simulink model "simulacion_ROS"  (R2025b)
settings: Solver=ode14x  StartTime=0.0  StopTime=20  FixedStep=0.01  RelTol=1e-3
InitFcn:
  | start_time_epoch = posixtime(datetime('now'))-3600;
  | setenv('ROS_LOCALHOST_ONLY', '');
  | setenv('RMW_IMPLEMENTATION','rmw_cyclonedds_cpp')
values from neighbouring files (symbols this model uses):
  A = [zeros(2),        eye(2) ... (first row only)    [parametros_planta.m]
  B = [0;0;[M_bar\[1;0]]]    [parametros_planta.m]
  cc = 0.05    [parametros_planta.m]
  cp = 0.0005    [parametros_planta.m]
  g = 9.81    [parametros_planta.m]
  J = 0.0136    [parametros_planta.m]
  lcm = 0.17    [parametros_planta.m]
  M = mp + mc    (= 1.23)    [parametros_planta.m]
  mc = 1.12    [parametros_planta.m]
  mp = 0.11    [parametros_planta.m]
undefined symbols (not defined in the file or in its folder): K_lqr
libraries: ros2lib x2
settings Model: Creator=miguel  LastModifiedBy=miguel
settings SolverCC: EnableFixedStepZeroCrossing=on
settings OptimizationCC: DefaultParameterBehavior=Inlined  EnhancedBackFolding=on  PassReuseOutputArgsAs=Individual arguments  ZeroExternalMemoryAtStartup=off  ZeroInternalMemoryAtStartup=off  MaxStackSize=64  OptimizeBlockOrder=speed  DifferentSizesBufferReuse=on  OptimizationCustomize=off  EfficientTunableParamExpr=on
settings DebuggingCC: ParameterTunabilityLossMsg=error
settings HardwareCC: ProdBitPerLong=64.0  ProdHWDeviceType=Intel->x86-64 (Linux 64)  UseEmbeddedCoderFeatures=off
settings SFSimCC: MATLABDynamicMemAlloc=off
settings RTWCC: SystemTargetFile=ert.tlc  HardwareBoard=Robot Operating System 2 (ROS 2)  TLCOptions="-aInlineSetEventsForThisBaseRateFcn=TLC_FALSE -aSuppressMultiTaskScheduler=TLC_FALSE  -aRateBasedStepFcn=0"  TemplateMakefile=ert_default_tmf  Toolchain=Colcon Tools  TargetLang=C++  Description=Embedded Coder
settings CodeAppCC: ForceParamTrailComments=on  IgnoreCustomStorageClasses=off  OperatorAnnotations=on  SimulinkDataObjDesc=on  SFDataObjDesc=on  InsertBlockDesc=on
settings ERTTargetCC: ExtModeTransport=2.0  ExtModeStaticAlloc=on  ExtModeAutomaticAllocSize=off  ExtModeMexFile=ext_xcp  ExtModeIntrfLevel=Level2 - Open  RootIOFormat=Structure reference  CodeInterfacePackaging=C++ class  SupportNonInlinedSFcns=on

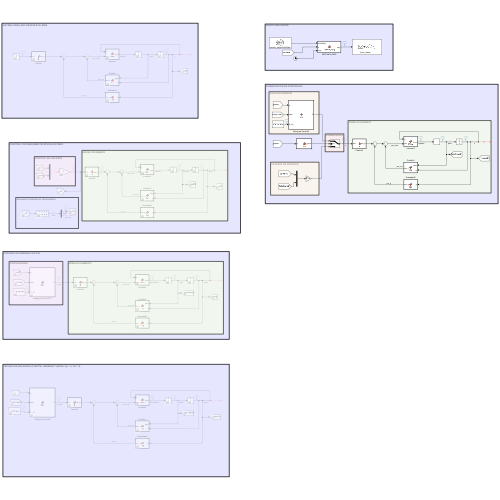
[thumbnail: Simulink's stored preview of the top-level diagram]
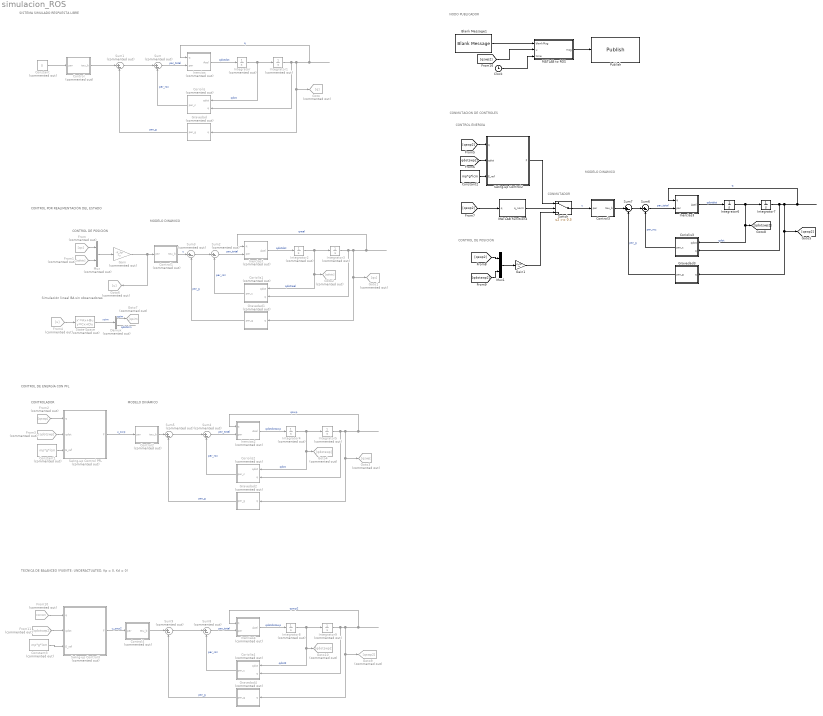
== system simulacion_ROS ==
  note: CONTROLADOR
  note: MODELO DINÁMICO
  note: CONTROL DE POSICIÓN
  note: MODELO DINÁMICO
  note: CONMUTADOR
  note: MODELO DINÁMICO
  note: CONTROL ENERGÍA
  note: CONTROL DE POSICIÓN
  note: Simulación lineal BA sin observadores
  note: SISTEMA SIMULADO RESPUESTA LIBRE
  note: NODO PUBLICADOR
  note: CONTROL POR REALIMENTACIÓN DEL ESTADO
  note: CONTROL DE ENERGÍA CON PFL
  note: CONMUTACION DE CONTROLES
  note: TECNICA DE BALANCEO (FUENTE: UNDERACTUATED, Kp = 0, Kd = 0)
  Blank Message1 : ros2lib/Blank Message  messageClass=Message  entityType=sensor_msgs/JointState  messageType=sensor_msgs/JointState  SampleTime=inf
  Clock : Clock
  Constant : Constant  Commented=on  Value=0
  Constant1 : Constant  Commented=on  Value=mp*g*lcm
  Constant2 : Constant  Value=mp*g*lcm
  Constant3 : Constant  Commented=on  Value=mp*g*lcm
  Control : MATLAB Function  Commented=on  TreatAsAtomicUnit=on
  Control1 : MATLAB Function  Commented=on  TreatAsAtomicUnit=on
  Control2 : MATLAB Function  Commented=on  TreatAsAtomicUnit=on
  Control3 : MATLAB Function  TreatAsAtomicUnit=on
  Control4 : MATLAB Function  Commented=on  TreatAsAtomicUnit=on
  Coriolis : MATLAB Function  Commented=on  TreatAsAtomicUnit=on
  Coriolis1 : MATLAB Function  Commented=on  TreatAsAtomicUnit=on
  Coriolis2 : MATLAB Function  Commented=on  TreatAsAtomicUnit=on
  Coriolis3 : MATLAB Function  TreatAsAtomicUnit=on
  Coriolis4 : MATLAB Function  Commented=on  TreatAsAtomicUnit=on
  Demux : Demux  Commented=on  Outputs=2
  From : From  Commented=on  GotoTag=qc
  From1 : From  Commented=on  GotoTag=qdotc
  From10 : From  Commented=on  GotoTag=qswp2
  From11 : From  Commented=on  GotoTag=qdotswp2
  From2 : From  Commented=on  GotoTag=qswp
  From3 : From  Commented=on  GotoTag=qdotswp
  From4 : From  Commented=on  GotoTag=u
  Gain : Gain  Commented=on  Gain=-K_lqr  Multiplication=Matrix(K*u)
  Gain1 : Gain  Gain=-K_lqr  Multiplication=Matrix(K*u)
  Goto : Goto  Commented=on  GotoTag=q
  Goto1 : Goto  Commented=on  GotoTag=qc
  Goto10 : Goto  Commented=on  GotoTag=qdotswp2
  Goto2 : Goto  Commented=on  GotoTag=qdotc
  Goto3 : Goto  Commented=on  GotoTag=qswp
  Goto4 : Goto  Commented=on  GotoTag=qdotswp
  Goto6 : Goto  Commented=on  GotoTag=u
  Goto7 : Goto  Commented=on  GotoTag=qsim
  Goto9 : Goto  Commented=on  GotoTag=qswp2
  Gravedad : MATLAB Function  Commented=on  TreatAsAtomicUnit=on
  Gravedad1 : MATLAB Function  Commented=on  TreatAsAtomicUnit=on
  Gravedad2 : MATLAB Function  Commented=on  TreatAsAtomicUnit=on
  Gravedad3 : MATLAB Function  TreatAsAtomicUnit=on
  Gravedad4 : MATLAB Function  Commented=on  TreatAsAtomicUnit=on
  Inercias : MATLAB Function  Commented=on  TreatAsAtomicUnit=on
  Inercias1 : MATLAB Function  Commented=on  TreatAsAtomicUnit=on
  Inercias2 : MATLAB Function  Commented=on  TreatAsAtomicUnit=on
  Inercias3 : MATLAB Function  TreatAsAtomicUnit=on
  Inercias4 : MATLAB Function  Commented=on  TreatAsAtomicUnit=on
  Integrator : Integrator  Commented=on  InitialCondition=[0; 0]
  Integrator1 : Integrator  Commented=on  InitialCondition=[0; 0.1]
  Integrator2 : Integrator  Commented=on  InitialCondition=[0; 0]
  Integrator3 : Integrator  Commented=on  InitialCondition=[0; 0.2]
  Integrator4 : Integrator  Commented=on  InitialCondition=[0; 0.01]
  Integrator5 : Integrator  Commented=on  InitialCondition=[0; 3.14]
  Integrator6 : Integrator  InitialCondition=[0; 0.01]
  Integrator7 : Integrator  InitialCondition=[0; 3.14]
  Integrator8 : Integrator  Commented=on  InitialCondition=[0; 0.01]
  Integrator9 : Integrator  Commented=on  InitialCondition=[0; 3.14]
  MATLAB Function4 : MATLAB Function  TreatAsAtomicUnit=on
  MATLAB to ROS : MATLAB Function  TreatAsAtomicUnit=on
  Mux : Mux  Commented=on  Inputs=2
  Mux1 : Mux  Inputs=2
  Publish : ros2lib/Publish  topicSource=Specify your own  topic=/joint_states  messageType=sensor_msgs/JointState  QOSHistory=Keep last  QOSDepth=10  QOSReliability=Reliable  QOSDurability=Volatile  QOSDeadline=Inf  QOSLifespan=Inf  QOSLiveliness=Automatic  QOSLeaseDuration=Inf  QOSAvoidROSNamespaceConventions=off
  State-Space : StateSpace  Commented=on  A=A  B=B  C=eye(4)  D=[0; 0; 0; 0]  InitialCondition=[0; 0.2; 0; 0]
  Sum{,1..5,8..9} (8 alike) : Sum  Commented=on  Inputs=|+-
  Sum6 : Sum  Inputs=|+-
  Sum7 : Sum  Inputs=|+-
  Swing-up Control PFL : MATLAB Function  Commented=on  TreatAsAtomicUnit=on
  Swing-up Control2 : MATLAB Function  TreatAsAtomicUnit=on
  Swing-up Control3 : MATLAB Function  Commented=on  TreatAsAtomicUnit=on
  Switch : Switch  Threshold=0.3  SaturateOnIntegerOverflow=off  InputSameDT=off
  wires:
  Sum1/1 -> Sum/1
  Gravedad/1(par_g) -> Sum1/2  "par_g"
  Control/1(tau_b) -> Sum1/1
  Integrator1/1 -> Coriolis/2(q), Goto/1, Gravedad/1(q), Inercias/1(q)  "q"
  Inercias/1(Acel) -> Integrator/1  "qdotdot"
  Constant/1 -> Control/1(par)
  Integrator/1 -> Coriolis/1(qdot), Integrator1/1  "qdot"
  Sum/1 -> Inercias/2(par)  "par_total"
  Coriolis/1(par_c) -> Sum/2  "par_roz"
  Blank Message1/1 -> MATLAB to ROS/1(blankMsg)
  MATLAB to ROS/1(msg) -> Publish/1
  Clock/1 -> MATLAB to ROS/3(time)
  [qswp2] -> MATLAB to ROS/2(u)
  Coriolis1/1(par_c) -> Sum2/2  "par_roz"
  Control1/1(tau_b) -> Sum3/1  "u"
  Integrator3/1 -> Coriolis1/2(q), Goto1/1, Gravedad1/1(q), Inercias1/1(q)  "qreal"
  Inercias1/1(Acel) -> Integrator2/1  "qdotdot"
  Sum2/1 -> Inercias1/2(par)  "par_total"
  Gravedad1/1(par_g) -> Sum3/2  "par_g"
  Sum3/1 -> Sum2/1
  Integrator2/1 -> Goto2/1, Coriolis1/1(qdot), Integrator3/1  "qdotreal"
  Mux/1 -> Gain/1
  From/1 -> Mux/1
  From1/1 -> Mux/2
  From4/1 -> State-Space/1
  State-Space/1 -> Demux/1  "xsim"
  Demux/1 -> Goto7/1  "qsim"
  Demux/2 -> ?  "qdotsim"
  Inercias2/1(Acel) -> Integrator4/1  "qdotdotswp"
  Integrator5/1 -> Coriolis2/2(q), Goto3/1, Gravedad2/1(q), Inercias2/1(q)  "qswp"
  Sum5/1 -> Sum4/1
  Gravedad2/1(par_g) -> Sum5/2  "par_g"
  Control2/1(tau_b) -> Sum5/1
  Integrator4/1 -> Goto4/1, Coriolis2/1(qdot), Integrator5/1  "qdot"
  Sum4/1 -> Inercias2/2(par)  "par_total"
  Coriolis2/1(par_c) -> Sum4/2  "par_roz"
  Swing-up Control PFL/1(F) -> Control2/1(par)  "u_swp"
  From2/1 -> Swing-up Control PFL/1(q)
  From3/1 -> Swing-up Control PFL/2(qdot)
  Constant2/1 -> Swing-up Control2/3(E_ref)
  Control3/1(tau_b) -> Sum7/1
  Coriolis3/1(par_c) -> Sum6/2  "par_roz"
  Sum7/1 -> Sum6/1
  Inercias3/1(Acel) -> Integrator6/1  "qdotdot"
  [qdotswp2] -> Swing-up Control2/2(qdot)
  Integrator6/1 -> [qdotswp2], Coriolis3/1(qdot), Integrator7/1  "qdot"
  Sum6/1 -> Inercias3/2(par)  "par_total"
  [qswp2] -> Swing-up Control2/1(q)
  Gravedad3/1(par_g) -> Sum7/2  "par_g"
  Integrator7/1 -> Coriolis3/2(q), [qswp2], Gravedad3/1(q), Inercias3/1(q)  "q"
  Switch/1 -> Control3/1(par)  "u"
  Swing-up Control2/1(F) -> Switch/1
  MATLAB Function4/1(q_norm) -> Switch/2
  [qswp2] -> MATLAB Function4/1(q)
  [qswp2] -> Mux1/1
  Mux1/1 -> Gain1/1
  [qdotswp2] -> Mux1/2
  Gain1/1 -> Switch/3
  Constant3/1 -> Swing-up Control3/3(E_ref)
  Control4/1(tau_b) -> Sum9/1
  Coriolis4/1(par_c) -> Sum8/2  "par_roz"
  Sum9/1 -> Sum8/1
  Inercias4/1(Acel) -> Integrator8/1  "qdotdotswp"
  From11/1 -> Swing-up Control3/2(qdot)
  Integrator8/1 -> Goto10/1, Coriolis4/1(qdot), Integrator9/1  "qdot2"
  Swing-up Control3/1(F) -> Control4/1(par)  "u_swp2"
  Sum8/1 -> Inercias4/2(par)  "par_total"
  From10/1 -> Swing-up Control3/1(q)
  Gravedad4/1(par_g) -> Sum9/2  "par_g"
  Integrator9/1 -> Coriolis4/2(q), Goto9/1, Gravedad4/1(q), Inercias4/1(q)  "qswp2"
  Constant1/1 -> Swing-up Control PFL/3(E_ref)
  Gain/1 -> Goto6/1, Control1/1(par)

== matlab function simulacion_ROS/Control2 ==
  data: par input; tau_b output
function tau_b = B(par)

tau_b = [1; 0]*par; %Nuestra acción de control se aplica sobre el eje horizontal.

== matlab function simulacion_ROS/Coriolis2 ==
  data: qdot input; q input; par_c output size=[2, 1]; cc parameter; cp parameter; mp parameter; lcm parameter
function par_c = Cq(qdot, q, cc, cp, mp, lcm)

%Nota: cp = 0 Nm.rad/s no me lo creo habrá que estimarlo de forma
%conservadora.

C = [cc,   -mp*lcm*qdot(2)*sin(q(2))
      0,          cp        ]; 

par_c = C*qdot;

== matlab function simulacion_ROS/Gravedad2 ==
  data: q input; par_g output; mp parameter; g parameter; lcm parameter
function par_g = Gq(q, mp, g, lcm)
G = [0; -mp*g*lcm*sin(q(2))]; 

par_g = G;

== matlab function simulacion_ROS/Inercias2 ==
  data: q input; par input; Acel output; J parameter; M parameter; mp parameter; lcm parameter
function Acel = Minv(q,par, J, M, mp, lcm)
%La matriz va aumentando su dimensionalidad a medida que se añaden GDLs

M = [M,          +mp*lcm*cos(q(2));
    +mp*lcm*cos(q(2)),      J]; 

Acel = M\par; %División de matrices.

== matlab function simulacion_ROS/Control3 ==
  data: par input; tau_b output
function tau_b = B(par)

tau_b = [1; 0]*par; %Nuestra acción de control se aplica sobre el eje horizontal.

== matlab function simulacion_ROS/Swing-up Control PFL ==
  data: q input; F output; qdot input; E_ref input; mp parameter; lcm parameter; cp parameter; cc parameter; J parameter; mc parameter
function F = fcn(q, qdot, E_ref, mp, lcm, cp, cc, J, mc) % Añadido Mc y salida F

% --- PARAMETROS FISICOS Y GANANCIAS ---
g = 9.81; % Añadido el punto y coma

% Ganancias del control de energía (Swing-up) AJUSTAR
Ke = 26; 
kp = 8.16; 
kd = 4; 

% -- ESTADOS DEL SISTEMA --
x = q(1);        % Posición del carro
theta = q(2);    % Ángulo del péndulo (0 = arriba)
xdot = qdot(1);  % Velocidad del carro
thetadot = qdot(2); % Velocidad angular

% --- 1. CÁLCULO DE ENERGÍA ---
Ep = mp * g * lcm * cos(theta); 
Ek = 0.5 * J * thetadot^2;
E_total = Ep + Ek;

% --- 2. LEY DE CONTROL DE ENERGÍA (Aceleración 'u') ---
e = E_total - E_ref;
u = Ke * thetadot * cos(theta) * e - kp * x - kd * xdot;

% --- 3. LINEARIZACIÓN POR RETROALIMENTACIÓN PARCIAL (PFL) ---
% Convierte la aceleración deseada 'u' en Fuerza 'F' para el motor

thetadotdot = 1/J *(-mp*lcm*cos(theta)*u ...
    + mp*g*lcm*sin(theta) -cp*thetadot);

F = (mc + mp) * u ...
    - (mp * lcm * thetadot^2 * sin(theta)) ...
    + (mp * lcm * cos(theta)) * thetadotdot ...
    +cc*xdot;

%Saturacion --> Evitar oscilaciones iniciales bruscas.
F_max = 2; % Newtons
if F > F_max
    F = F_max;
elseif F < -F_max
    F = -F_max;
end

end

== matlab function simulacion_ROS/Coriolis3 ==
  data: qdot input; q input; par_c output size=[2, 1]; cc parameter; cp parameter; mp parameter; lcm parameter
function par_c = Cq(qdot, q, cc, cp, mp, lcm)

%Nota: cp = 0 Nm.rad/s no me lo creo habrá que estimarlo de forma
%conservadora.

C = [cc,   -mp*lcm*qdot(2)*sin(q(2))
      0,          cp        ]; 

par_c = C*qdot;

== matlab function simulacion_ROS/Gravedad3 ==
  data: q input; par_g output; mp parameter; g parameter; lcm parameter
function par_g = Gq(q, mp, g, lcm)
G = [0; -mp*g*lcm*sin(q(2))]; 

par_g = G;

== matlab function simulacion_ROS/Inercias3 ==
  data: q input; par input; Acel output; J parameter; M parameter; mp parameter; lcm parameter
function Acel = Minv(q,par, J, M, mp, lcm)
%La matriz va aumentando su dimensionalidad a medida que se añaden GDLs

M = [M,          +mp*lcm*cos(q(2));
    +mp*lcm*cos(q(2)),      J]; 

Acel = M\par; %División de matrices.

== matlab function simulacion_ROS/Swing-up Control2 ==
  data: q input; F output; qdot input; E_ref input; mp parameter; lcm parameter; cp parameter; cc parameter; J parameter; mc parameter
function F = fcn(q, qdot, E_ref, mp, lcm, cp, cc, J, mc) 

% --- PARAMETROS FISICOS Y GANANCIAS ---
g = 9.81; 

% Ganancias del control de energía (Swing-up)
Ke = 26; 
kp = 6; 
kd = 4; 

% -- ESTADOS DEL SISTEMA --
x = q(1);        % Posición del carro
theta = q(2);    % Ángulo del péndulo 
xdot = qdot(1);  % Velocidad del carro
thetadot = qdot(2); % Velocidad angular

% --- 1. CÁLCULO DE ENERGÍA ---
Ep = mp * g * lcm * cos(theta); 
Ek = 0.5 * J * thetadot^2;
E_total = Ep + Ek;

% --- 2. LEY DE CONTROL DE ENERGÍA (Aceleración 'u') ---
e = E_total - E_ref;
u = Ke * thetadot * cos(theta) * e - kp * x - kd * xdot;

% --- 3. LINEARIZACIÓN POR RETROALIMENTACIÓN PARCIAL (PFL) ---
% Convierte la aceleración deseada 'u' en Fuerza 'F' para el motor

thetadotdot = 1/J *(-mp*lcm*cos(theta)*u ...
    + mp*g*lcm*sin(theta) -cp*thetadot);

F = (mc + mp) * u ...
    - (mp * lcm * thetadot^2 * sin(theta)) ...
    + (mp * lcm * cos(theta)) * thetadotdot ...
    +cc*xdot;

%Saturacion --> Evitar oscilaciones iniciales bruscas.
F_max = 2; % Newtons
if F > F_max
    F = F_max;
elseif F < -F_max
    F = -F_max;
end

end

== matlab function simulacion_ROS/Coriolis ==
  data: qdot input; q input; par_c output size=[2, 1]; cc parameter; cp parameter; mp parameter; lcm parameter
function par_c = Cq(qdot, q, cc, cp, mp, lcm)

%Nota: cp = 0 Nm.rad/s no me lo creo habrá que estimarlo de forma
%conservadora.

C = [cc,   -mp*lcm*qdot(2)*sin(q(2))
      0,          cp        ]; 

par_c = C*qdot;

== matlab function simulacion_ROS/MATLAB Function4 ==
  data: q input; q_norm output
function q_norm = fcn(q)
    % Esto envuelve el ángulo para que siempre esté entre -pi y +pi
    q_norm = atan2(sin(q(2)), cos(q(2)));
    q_norm = abs(q_norm);
end

== matlab function simulacion_ROS/MATLAB to ROS ==
  data: blankMsg input; msg output Bus: SL_Bus_sensor_msgs_JointState; u input; time input; start_time_epoch parameter
function msg = create_msg(blankMsg, u, time, start_time_epoch)
%#codegen
msg = blankMsg;

%Sincronización con el reloj interno de la máquina.
total_time = start_time_epoch + time; 
%Indicar el tiempo de simulación para que RViz pueda componer la
%simulación. 
s = floor(total_time);
ns = (total_time - s) * 1e9;  
msg.header.stamp.sec = int32(s);
msg.header.stamp.nanosec = uint32(ns);

% Definimos los nombres y sus posiciones correspondientes
strArrayToAssign = {'cart_slider', 'pole_joint'};
% Las posiciones angulares de nuestro péndulo. 
positionsToAssign = [u(1), u(2)]; 

% 1. Configurar NOMBRES (Strings)
numStringsInArray = length(strArrayToAssign);
msg.name_SL_Info.CurrentLength = uint32(numStringsInArray);

for idx=1:numStringsInArray
    str = strArrayToAssign{idx};
    strLength = length(str);
    % Asignar caracteres convertidos a uint8
    msg.name(idx).data(1:strLength) = uint8(str);
    msg.name(idx).data_SL_Info.CurrentLength = uint32(strLength);
end

% 2. Configurar POSICIONES (float64 array)
% El campo 'position' en un Bus de Simulink para JointState 
% también tiene un campo _SL_Info asociado para controlar la longitud.
numPositions = length(positionsToAssign);
msg.position_SL_Info.CurrentLength = uint32(numPositions);
% Asignamos los valores directamente
msg.position(1:numPositions) = positionsToAssign;

% 3. Dejar sin campo de velocidad y esfuerzo el tópico.
msg.velocity_SL_Info.CurrentLength = uint32(0);
msg.effort_SL_Info.CurrentLength = uint32(0);

end

== matlab function simulacion_ROS/Control4 ==
  data: par input; tau_b output
function tau_b = B(par)

tau_b = [1; 0]*par; %Nuestra acción de control se aplica sobre el eje horizontal.

== matlab function simulacion_ROS/Coriolis4 ==
  data: qdot input; q input; par_c output size=[2, 1]; cc parameter; cp parameter; mp parameter; lcm parameter
function par_c = Cq(qdot, q, cc, cp, mp, lcm)

%Nota: cp = 0 Nm.rad/s no me lo creo habrá que estimarlo de forma
%conservadora.

C = [cc,   -mp*lcm*qdot(2)*sin(q(2))
      0,          cp        ]; 

par_c = C*qdot;

== matlab function simulacion_ROS/Gravedad4 ==
  data: q input; par_g output; mp parameter; g parameter; lcm parameter
function par_g = Gq(q, mp, g, lcm)
G = [0; -mp*g*lcm*sin(q(2))]; 

par_g = G;

== matlab function simulacion_ROS/Inercias4 ==
  data: q input; par input; Acel output; J parameter; M parameter; mp parameter; lcm parameter
function Acel = Minv(q,par, J, M, mp, lcm)
%La matriz va aumentando su dimensionalidad a medida que se añaden GDLs

M = [M,          +mp*lcm*cos(q(2));
    +mp*lcm*cos(q(2)),      J]; 

Acel = M\par; %División de matrices.

== matlab function simulacion_ROS/Swing-up Control3 ==
  data: q input; F output; qdot input; E_ref input; mp parameter; lcm parameter; cp parameter; cc parameter; J parameter; mc parameter
function F = fcn(q, qdot, E_ref, mp, lcm, cp, cc, J, mc) % Añadido Mc y salida F

% --- PARAMETROS FISICOS Y GANANCIAS ---
g = 9.81; % Añadido el punto y coma

% Ganancias del control de energía (Swing-up) AJUSTAR
Ke = 4; 
kp = 1.77; 
kd = 2.66; 

% -- ESTADOS DEL SISTEMA --
x = q(1);        % Posición del carro
theta = q(2);    % Ángulo del péndulo (0 = arriba)
xdot = qdot(1);  % Velocidad del carro
thetadot = qdot(2); % Velocidad angular

% --- 1. CÁLCULO DE ENERGÍA ---
Ep = mp * g * lcm * cos(theta); 
Ek = 0.5 * J * thetadot^2;
E_total = Ep + Ek;

% --- 2. LEY DE CONTROL DE ENERGÍA (Aceleración 'u') ---
e = E_total - E_ref;
u = Ke * thetadot * cos(theta) * e ;%- kp * x - kd * xdot;

% --- 3. LINEARIZACIÓN POR RETROALIMENTACIÓN PARCIAL (PFL) ---
% Convierte la aceleración deseada 'u' en Fuerza 'F' para el motor

thetadotdot = 1/J *(-mp*lcm*cos(theta)*u ...
    + mp*g*lcm*sin(theta) -cp*thetadot);

F = (mc + mp) * u ...
    - (mp * lcm * thetadot^2 * sin(theta)) ...
    + (mp * lcm * cos(theta)) * thetadotdot ...
    +cc*xdot;

% Opcional: Saturación de la fuerza para no quemar el motor
F_max = 18; % Newtons
if F > F_max
    F = F_max;
elseif F < -F_max
    F = -F_max;
end

end

== matlab function simulacion_ROS/Inercias ==
  data: q input; par input; Acel output; J parameter; M parameter; mp parameter; lcm parameter
function Acel = Minv(q,par, J, M, mp, lcm)
%La matriz va aumentando su dimensionalidad a medida que se añaden GDLs

M = [M,          +mp*lcm*cos(q(2));
    +mp*lcm*cos(q(2)),      J]; 

Acel = M\par; %División de matrices.

== matlab function simulacion_ROS/Gravedad ==
  data: q input; par_g output; mp parameter; g parameter; lcm parameter
function par_g = Gq(q, mp, g, lcm)
G = [0; -mp*g*lcm*sin(q(2))]; 

par_g = G;

== matlab function simulacion_ROS/Control ==
  data: par input; tau_b output
function tau_b = B(par)

tau_b = [1; 0]*par; %Nuestra acción de control se aplica sobre el eje horizontal.

== matlab function simulacion_ROS/Control1 ==
  data: par input; tau_b output
function tau_b = B(par)

tau_b = [1; 0]*par; %Nuestra acción de control se aplica sobre el eje horizontal.

== matlab function simulacion_ROS/Coriolis1 ==
  data: qdot input; q input; par_c output size=[2, 1]; cc parameter; cp parameter; mp parameter; lcm parameter
function par_c = Cq(qdot, q, cc, cp, mp, lcm)

%Nota: cp = 0 Nm.rad/s no me lo creo habrá que estimarlo de forma
%conservadora.

C = [cc,   -mp*lcm*qdot(2)*sin(q(2))
      0,          cp        ]; 

par_c = C*qdot;

== matlab function simulacion_ROS/Gravedad1 ==
  data: q input; par_g output; mp parameter; g parameter; lcm parameter
function par_g = Gq(q, mp, g, lcm)
G = [0; -mp*g*lcm*sin(q(2))]; 

par_g = G;

== matlab function simulacion_ROS/Inercias1 ==
  data: q input; par input; Acel output; J parameter; M parameter; mp parameter; lcm parameter
function Acel = Minv(q,par, J, M, mp, lcm)
%La matriz va aumentando su dimensionalidad a medida que se añaden GDLs

M = [M,          +mp*lcm*cos(q(2));
    +mp*lcm*cos(q(2)),      J]; 

Acel = M\par; %División de matrices.
